simulink model "sqr_pls_fourier"  (R2022b)
settings: Solver=VariableStepAuto  StartTime=0.0  StopTime=10.0  RelTol=1e-3
settings Model: Creator=metal  LastModifiedBy=metal

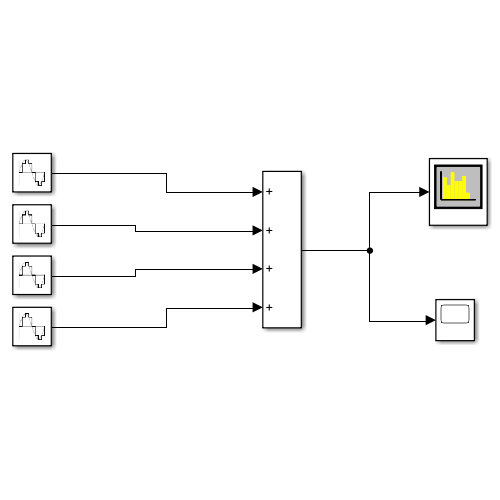
[thumbnail: Simulink's stored preview of the top-level diagram]
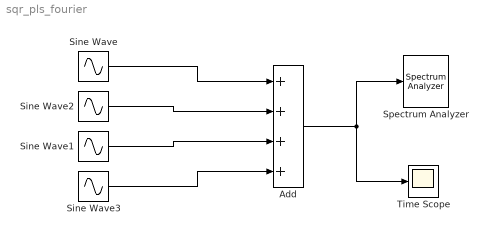
== system sqr_pls_fourier ==
  Add : Sum  Inputs=++++
  Sine Wave : Sin  Frequency=100  SampleTime=1/1024
  Sine Wave1 : Sin  Amplitude=1/3  Frequency=500  SampleTime=1/1024
  Sine Wave2 : Sin  Amplitude=1/3  Frequency=300  SampleTime=1/1024
  Sine Wave3 : Sin  Amplitude=1/3  Frequency=700  SampleTime=1/1024
  Spectrum Analyzer : SpectrumAnalyzer
  Time Scope : Scope
  wires:
  Sine Wave/1 -> Add/1
  Sine Wave2/1 -> Add/2
  Sine Wave1/1 -> Add/3
  Sine Wave3/1 -> Add/4
  Add/1 -> Spectrum Analyzer/1, Time Scope/1
